simulink model "two_para_adaptive_learning"  (R2016b)
settings: Solver=VariableStepAuto  StartTime=0.0  StopTime=100  RelTol=1e-3
libraries: simulink x1
settings Model: Creator=sxh  LastModifiedBy=sxh

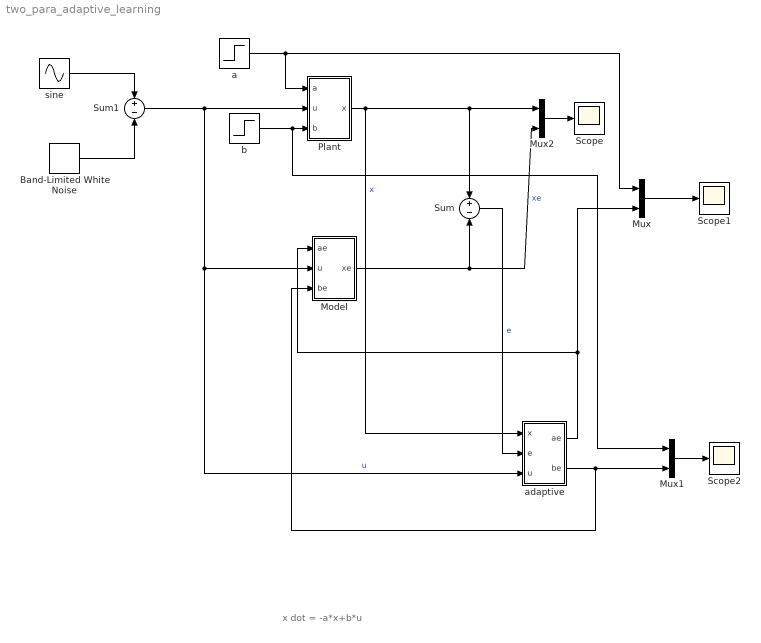
== system two_para_adaptive_learning ==
  note: x dot = -a*x+b*u
  Band-Limited White Noise : simulink/Sources/Band-Limited White Noise  Cov=1  Ts=0.1  seed=[23341]
  Model : Subsystem
  Mux : Mux  Inputs=2
  Mux1 : Mux  Inputs=2
  Mux2 : Mux  Inputs=2
  Plant : Subsystem
  Scope : Scope
  Scope1 : Scope
  Scope2 : Scope
  Sum : Sum  Inputs=+-
  Sum1 : Sum  Inputs=+-
  a : Step  Time=50  Before=2  After=4  SampleTime=0
  "adaptive " : Subsystem
  b : Step  Time=50  Before=1  After=3  SampleTime=0
  sine : Sin  Bias=5  Frequency=0.2  SampleTime=0
  wires:
  a/1 -> Mux/1, Plant/1(a)
  Plant/1(x) -> "adaptive "/1(x), Mux2/1, Sum/1  "x"
  Model/1(xe) -> Mux2/2, Sum/2  "xe"
  Mux/1 -> Scope1/1
  b/1 -> Mux1/1, Plant/3(b)
  Mux1/1 -> Scope2/1
  Mux2/1 -> Scope/1
  sine/1 -> Sum1/1
  Sum1/1 -> "adaptive "/3(u), Model/2(u), Plant/2(u)  "u"
  Band-Limited White Noise/1 -> Sum1/2
  "adaptive "/1(ae) -> Mux/2, Model/1(ae)
  "adaptive "/2(be) -> Model/3(be), Mux1/2
  Sum/1 -> "adaptive "/2(e)  "e"

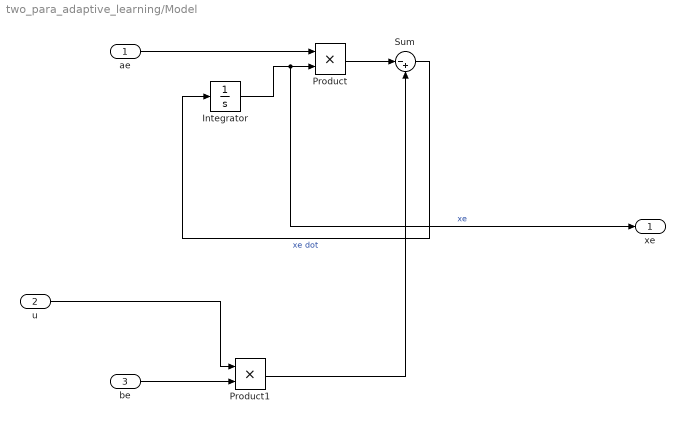
== system two_para_adaptive_learning/Model ==
  ae : Inport
  u : Inport  Port=2
  be : Inport  Port=3
  Integrator : Integrator  InitialCondition=9
  Product : Product
  Product1 : Product
  Sum : Sum  Inputs=|-+
  xe : Outport
  wires:
  ae/1 -> Product/1
  u/1 -> Product1/1
  Product1/1 -> Sum/2
  be/1 -> Product1/2
  Sum/1 -> Integrator/1  "xe dot"
  Integrator/1 -> xe/1, Product/2  "xe"
  Product/1 -> Sum/1

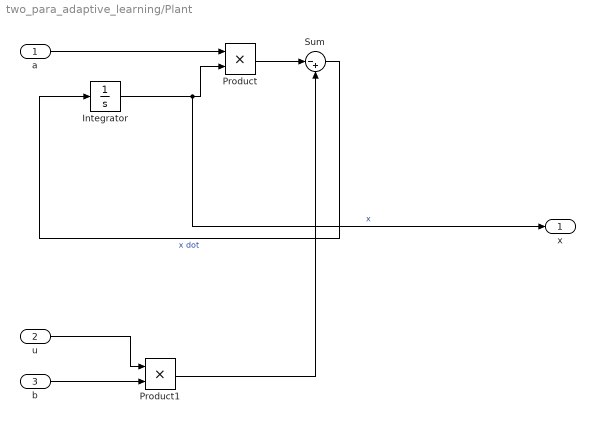
== system two_para_adaptive_learning/Plant ==
  a : Inport
  u : Inport  Port=2
  b : Inport  Port=3
  Integrator : Integrator  InitialCondition=10
  Product : Product
  Product1 : Product
  Sum : Sum  Inputs=|-+
  x : Outport
  wires:
  a/1 -> Product/1
  u/1 -> Product1/1
  Product1/1 -> Sum/2
  b/1 -> Product1/2
  Sum/1 -> Integrator/1  "x dot"
  Product/1 -> Sum/1
  Integrator/1 -> x/1, Product/2  "x"

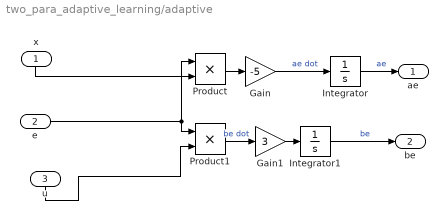
== system two_para_adaptive_learning/adaptive  ==
  x : Inport
  e : Inport  Port=2
  u : Inport  Port=3
  Gain : Gain  Gain=-5
  Gain1 : Gain  Gain=3
  Integrator : Integrator  InitialCondition=2
  Integrator1 : Integrator  InitialCondition=1
  Product : Product
  Product1 : Product
  ae : Outport
  be : Outport  Port=2
  wires:
  Gain1/1 -> Integrator1/1
  Gain/1 -> Integrator/1  "ae dot"
  Integrator1/1 -> be/1  "be"
  Product1/1 -> Gain1/1  "be dot"
  Integrator/1 -> ae/1  "ae"
  e/1 -> Product/1, Product1/1
  Product/1 -> Gain/1
  x/1 -> Product/2
  u/1 -> Product1/2
